simulink model "tir_model"  (Simulink 7.6)
settings: Solver=ode45  StartTime=0.0  StopTime=100  RelTol=1e-3
values from neighbouring files (symbols this model uses):
  ct10 = 27627    [semi_trailer.m]
  ct11 = 0    [semi_trailer.m]
  ct12 = 27627    [semi_trailer.m]
  ct13 = 0    [semi_trailer.m]
  ct14 = 27627    [semi_trailer.m]
  ct15 = 0    [semi_trailer.m]
  ct16 = 27627    [semi_trailer.m]
  ct17 = 0    [semi_trailer.m]
  ct18 = 10000    [semi_trailer.m]
  ct19 = 0    [semi_trailer.m]
  ct2 = 44506    [semi_trailer.m]
  ct20 = 10000    [semi_trailer.m]
  ct21 = 0    [semi_trailer.m]
  ct4 = 44506    [semi_trailer.m]
  ct6 = 44506    [semi_trailer.m]
  ct8 = 44506    [semi_trailer.m]
  dyt = 0.007    [semi_trailer.m]
  kt10 = 967430    [semi_trailer.m]
  kt11 = 2000000    [semi_trailer.m]
  kt12 = 967430    [semi_trailer.m]
  kt13 = 2000000    [semi_trailer.m]
  kt14 = 967430    [semi_trailer.m]
  kt15 = 2000000    [semi_trailer.m]
  kt16 = 967430    [semi_trailer.m]
  kt17 = 2000000    [semi_trailer.m]
  kt18 = 300000    [semi_trailer.m]
  kt19 = 847000    [semi_trailer.m]
  kt2 = 155800    [semi_trailer.m]
  kt20 = 300000    [semi_trailer.m]
  kt21 = 847000    [semi_trailer.m]
  kt3 = 2000000    [semi_trailer.m]
  kt4 = 155800    [semi_trailer.m]
  kt5 = 2000000    [semi_trailer.m]
  kt6 = 155800    [semi_trailer.m]
  kt7 = 2000000    [semi_trailer.m]
  kt8 = 155800    [semi_trailer.m]
  kt9 = 2000000    [semi_trailer.m]
  Lt11 = 4.8    [semi_trailer.m]
  Lt12 = 1.2    [semi_trailer.m]
  Lt13 = 3.6    [semi_trailer.m]
  Lt14 = 1.2    [semi_trailer.m]
  Lt15 = 1.2    [semi_trailer.m]
  Lt16 = 4.134    [semi_trailer.m]
  Lt21 = 4    [semi_trailer.m]
  Lt22 = 0.685    [semi_trailer.m]
  Lt23 = 0.7    [semi_trailer.m]
  Lt24 = 1.2    [semi_trailer.m]
  Lt25 = 1.2    [semi_trailer.m]
  Lt26 = 6.973    [semi_trailer.m]
  mt10 = 520    [semi_trailer.m]
  mt11 = 270    [semi_trailer.m]
  mt12 = 270    [semi_trailer.m]
  mt3 = 270    [semi_trailer.m]
  mt4 = 270    [semi_trailer.m]
  mt5 = 270    [semi_trailer.m]
  mt6 = 270    [semi_trailer.m]
  mt7 = 520    [semi_trailer.m]
  mt8 = 520    [semi_trailer.m]
  mt9 = 520    [semi_trailer.m]
  Vt = 20    [semi_trailer.m]
  wt = 20/dyt    (= 2857.14285714)    [semi_trailer.m]
settings Model: Creator=user  LastModifiedBy=user

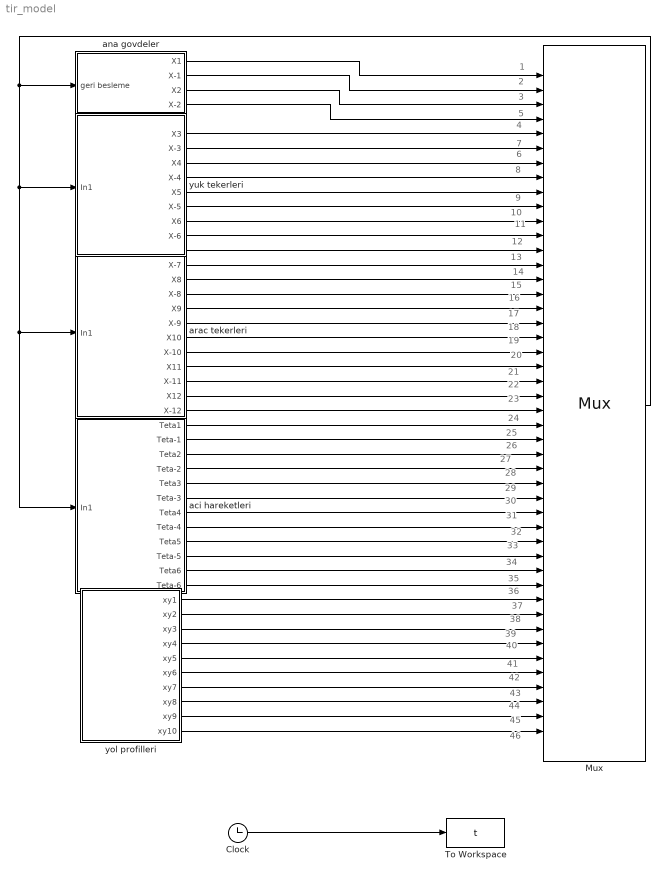
== system tir_model ==
  note: 1
  note: 2
  note: 3
  note: 4
  note: 5
  note: 6
  note: 7
  note: 8
  note: 9
  note: 10
  note: 11
  note: 12
  note: 13
  note: 14
  note: 15
  note: 16
  note: 17
  note: 18
  note: 19
  note: 20
  note: 21
  note: 22
  note: 23
  note: 24
  note: 25
  note: 26
  note: 27
  note: 28
  note: 29
  note: 30
  note: 31
  note: 32
  note: 33
  note: 34
  note: 35
  note: 36
  note: 37
  note: 38
  note: 39
  note: 40
  note: 41
  note: 42
  note: 43
  note: 44
  note: 45
  note: 46
  Clock : Clock
      settings: Decimation=10
  Mux : Mux  Inputs=46
  To Workspace : ToWorkspace  VariableName=t  SampleTime=-1  SaveFormat=Array
  aci hareketleri : Subsystem
  ana govdeler : Subsystem
  arac tekerleri : Subsystem
  yol profilleri : Subsystem
  "yuk tekerleri " : Subsystem
  wires:
  Clock/1 -> To Workspace/1
  "yuk tekerleri "/1(X3) -> Mux/5
  "yuk tekerleri "/2(X-3) -> Mux/6
  "yuk tekerleri "/3(X4) -> Mux/7
  "yuk tekerleri "/4(X-4) -> Mux/8
  "yuk tekerleri "/5(X5) -> Mux/9
  "yuk tekerleri "/6(X-5) -> Mux/10
  "yuk tekerleri "/7(X6) -> Mux/11
  "yuk tekerleri "/8(X-6) -> Mux/12
  arac tekerleri/1(X7) -> Mux/13
  arac tekerleri/2(X-7) -> Mux/14
  arac tekerleri/3(X8) -> Mux/15
  arac tekerleri/4(X-8) -> Mux/16
  arac tekerleri/5(X9) -> Mux/17
  arac tekerleri/6(X-9) -> Mux/18
  arac tekerleri/7(X10) -> Mux/19
  arac tekerleri/8(X-10) -> Mux/20
  arac tekerleri/9(X11) -> Mux/21
  arac tekerleri/10(X-11) -> Mux/22
  arac tekerleri/11(X12) -> Mux/23
  arac tekerleri/12(X-12) -> Mux/24
  aci hareketleri/1(Teta1) -> Mux/25
  aci hareketleri/2(Teta-1) -> Mux/26
  aci hareketleri/3(Teta2) -> Mux/27
  aci hareketleri/4(Teta-2) -> Mux/28
  aci hareketleri/5(Teta3) -> Mux/29
  aci hareketleri/6(Teta-3) -> Mux/30
  aci hareketleri/7(Teta4) -> Mux/31
  aci hareketleri/8(Teta-4) -> Mux/32
  aci hareketleri/9(Teta5) -> Mux/33
  aci hareketleri/10(Teta-5) -> Mux/34
  aci hareketleri/11(Teta6) -> Mux/35
  aci hareketleri/12(Teta-6) -> Mux/36
  Mux/1 -> aci hareketleri/1(In1), arac tekerleri/1(In1), "yuk tekerleri "/1(In1), ana govdeler/1(geri besleme)
  ana govdeler/1(X1) -> Mux/1
  ana govdeler/2(X-1) -> Mux/2
  ana govdeler/3(X2) -> Mux/3
  ana govdeler/4(X-2) -> Mux/4
  yol profilleri/1(xy1) -> Mux/37
  yol profilleri/2(xy2) -> Mux/38
  yol profilleri/3(xy3) -> Mux/39
  yol profilleri/4(xy4) -> Mux/40
  yol profilleri/5(xy5) -> Mux/41
  yol profilleri/6(xy6) -> Mux/42
  yol profilleri/7(xy7) -> Mux/43
  yol profilleri/8(xy8) -> Mux/44
  yol profilleri/9(xy9) -> Mux/45
  yol profilleri/10(xy10) -> Mux/46

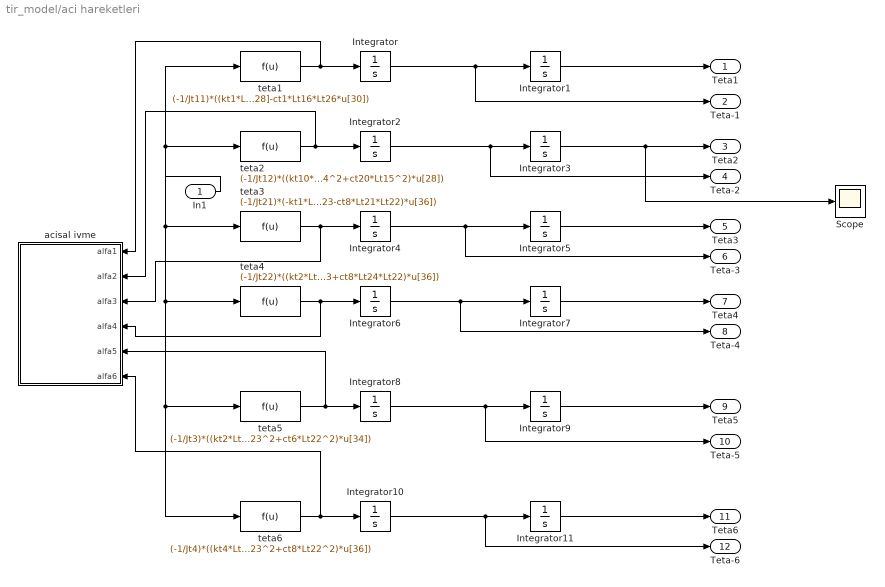
== system tir_model/aci hareketleri ==
  In1 : Inport
  Integrator{,1..11} (12 alike) : Integrator
  Scope : Scope
      settings: SaveName=ScopeData2
  acisal ivme : Subsystem
  teta1 : Fcn  Expr=(-1/Jt11)*((kt1*Lt16+kt10*Lt11+kt12*Lt11+kt14*Lt13+kt16*Lt13-kt18*Lt12-kt20*Lt12)*u[1]+kt1*Lt16*u[3]-kt10*Lt11*u[13]-kt12*Lt11*u[15]-kt14*Lt13*u[17]-kt16*Lt13*u[19]+kt18*Lt12*u[21]+kt20*Lt12*u[23]+(kt1*Lt16^2+kt10*Lt11^2+kt12*Lt11^2+kt14*Lt13^2+kt16*Lt13^2+kt18*Lt12^2+kt20*Lt12^2)*u[25]+(kt10*Lt11*Lt14-kt12*Lt11*Lt15+kt14*Lt13*Lt14-kt16*Lt13*Lt15-kt18*Lt12*Lt14+kt20*Lt12*Lt15)*u[27]-kt1*Lt16*Lt26*u[29]+(ct1*Lt16+ct10*Lt11+ct12*Lt11+ct14*Lt13+ct16*Lt13-ct18*Lt12-ct20*Lt12)*u[2]+ct1*Lt16*u[4]-ct10*Lt11*u[14]-ct12*Lt11*u[16]-ct14*Lt13*u[18]-ct16*Lt13*u[20]+ct18*Lt12*u[22]+ct20*Lt12*u[24]+(ct1*Lt16^2+ct10*Lt11^2+ct12*Lt11^2+ct14*Lt13^2+ct16*Lt13^2+ct18*Lt12^2+ct20*Lt12^2)*u[26]+(ct10*Lt11*Lt14-ct12*Lt11*Lt15+ct14*Lt13*Lt14-ct16*Lt13*Lt15-ct18*Lt12*Lt14+ct20*Lt12*Lt15)*u[28]-ct1*Lt16*Lt26*u[30])
  teta2 : Fcn  Expr=(-1/Jt12)*((kt10*Lt14-kt12*Lt15+kt14*Lt14-kt16*Lt15+kt18*Lt14-kt20*Lt15)*u[1]-kt10*Lt14*u[13]+kt12*Lt15*u[15]-kt14*Lt14*u[17]+kt16*Lt15*u[19]-kt18*Lt14*u[21]+kt20*Lt15*u[23]+(kt10*Lt11*Lt14-kt12*Lt11*Lt15+kt14*Lt13*Lt14-kt16*Lt13*Lt15-kt18*Lt12*Lt14+kt20*Lt12*Lt15)*u[25]+(kt10*Lt14^2+kt12*Lt15^2+kt14*Lt14^2+kt16*Lt15^2+kt18*Lt14^2+kt20*Lt15^2)*u[27]+(ct10*Lt14-ct12*Lt15+ct14*Lt14-ct16*Lt15+ct18*Lt14-ct20*Lt15)*u[2]-ct10*Lt14*u[14]+ct12*Lt15*u[16]-ct14*Lt14*u[18]+ct16*Lt15*u[20]-ct18*Lt14*u[22]+ct20*Lt15*u[24]+(ct10*Lt11*Lt14-ct12*Lt11*Lt15+ct14*Lt13*Lt14-ct16*Lt13*Lt15-ct18*Lt12*Lt14+ct20*Lt12*Lt15)*u[26]+(ct10*Lt14^2+ct12*Lt15^2+ct14*Lt14^2+ct16*Lt15^2+ct18*Lt14^2+ct20*Lt15^2)*u[28])
  teta3 : Fcn  Expr=(-1/Jt21)*(-kt1*Lt26*u[1]+(-kt1*Lt26+kt2*Lt21+kt4*Lt21+kt6*Lt21+kt8*Lt21)*u[3]-kt2*Lt21*u[5]-kt4*Lt21*u[7]-kt6*Lt21*u[9]-kt8*Lt21*u[11]-kt1*Lt16*Lt26*u[25]+(kt1*Lt26^2+kt2*Lt21^2+kt4*Lt21^2+kt6*Lt21^2+kt8*Lt21^2)*u[29]+(kt2*Lt21*Lt24-kt4*Lt21*Lt25+kt6*Lt21*Lt24-kt8*Lt21*Lt25)*u[31]+(kt2*Lt21*Lt23-kt6*Lt21*Lt22)*u[33]+(kt4*Lt21*Lt23-kt8*Lt21*Lt22)*u[35]-ct1*Lt26*u[2]+(-ct1*Lt26+ct2*Lt21+ct4*Lt21+ct6*Lt21+ct8*Lt21)*u[4]-ct2*Lt21*u[6]-ct4*Lt21*u[8]-ct6*Lt21*u[10]-ct8*Lt21*u[12]-ct1*Lt16*Lt26*u[26]+(ct1*Lt26^2+ct2*Lt21^2+ct4*Lt21^2+ct6*Lt21^2+ct8*Lt21^2)*u[30]+(ct2*Lt21*Lt24-ct4*Lt21*Lt25+ct6*Lt21*Lt24-ct8*Lt21*Lt25)*u[32]+(ct2*Lt21*Lt23-ct6*Lt21*Lt22)*u[34]+(ct4*Lt21*Lt23-ct8*Lt21*Lt22)*u[36])
  teta4 : Fcn  Expr=(-1/Jt22)*((kt2*Lt24-kt4*Lt25+kt6*Lt24-kt8*Lt25)*u[3]-kt2*Lt24*u[5]+kt4*Lt25*u[7]-kt6*Lt24*u[9]+kt8*Lt25*u[11] +(kt2*Lt21*Lt24-kt4*Lt21*Lt25+kt6*Lt21*Lt24-kt8*Lt21*Lt25)*u[29]+(kt2*Lt24^2+kt4*Lt25^2+kt6*Lt24^2+kt8*Lt25^2)*u[31]+(kt2*Lt24*Lt23-kt6*Lt24*Lt22)*u[33]+(-kt4*Lt25*Lt23+kt8*Lt24*Lt22)*u[35]+(ct2*Lt24-ct4*Lt25+ct6*Lt24-ct8*Lt25)*u[4]-ct2*Lt24*u[6]+ct4*Lt25*u[8]-ct6*Lt24*u[10]+ct8*Lt25*u[12]+(ct2*Lt21*Lt24-ct4*Lt21*Lt25+ct6*Lt21*Lt24-ct8*Lt21*Lt25)*u[30]+(ct2*Lt24^2+ct4*Lt25^2+ct6*Lt24^2+ct8*Lt25^2)*u[32]+(ct2*Lt24*Lt23-ct6*Lt24*Lt22)*u[34]+(-ct4*Lt25*Lt23+ct8*Lt24*Lt22)*u[36])
  teta5 : Fcn  Expr=(-1/Jt3)*((kt2*Lt23-kt6*Lt22)*u[3]-kt2*Lt23*u[5]+kt6*Lt22*u[9]+(kt2*Lt23*Lt21-kt6*Lt22*Lt21)*u[29]+(kt2*Lt23*Lt24-kt6*Lt22*Lt24)*u[31]+(kt2*Lt23^2+kt6*Lt22^2)*u[33]+(ct2*Lt23-ct6*Lt22)*u[4]-ct2*Lt23*u[6]+ct6*Lt22*u[10]+(ct2*Lt23*Lt21-ct6*Lt22*Lt21)*u[30]+(ct2*Lt23*Lt24-ct6*Lt22*Lt24)*u[32]+(ct2*Lt23^2+ct6*Lt22^2)*u[34])
  teta6 : Fcn  Expr=(-1/Jt4)*((kt4*Lt23-kt8*Lt22)*u[3]-kt4*Lt23*u[7]+kt8*Lt22*u[11]+(kt4*Lt23*Lt21-kt8*Lt22*Lt21)*u[29]+(-kt4*Lt23*Lt25+kt8*Lt22*Lt25)*u[31]+(kt4*Lt23^2+kt8*Lt22^2)*u[35]+(ct4*Lt23-ct8*Lt22)*u[4]-ct4*Lt23*u[8]+ct8*Lt22*u[12]+(ct4*Lt23*Lt21-ct8*Lt22*Lt21)*u[30]+(-ct4*Lt23*Lt25+ct8*Lt22*Lt25)*u[32]+(ct4*Lt23^2+ct8*Lt22^2)*u[36])
  Teta1 : Outport
  Teta-1 : Outport  Port=2
  Teta2 : Outport  Port=3
  Teta-2 : Outport  Port=4
  Teta3 : Outport  Port=5
  Teta-3 : Outport  Port=6
  Teta4 : Outport  Port=7
  Teta-4 : Outport  Port=8
  Teta5 : Outport  Port=9
  Teta-5 : Outport  Port=10
  Teta6 : Outport  Port=11
  Teta-6 : Outport  Port=12
  wires:
  Integrator10/1 -> Integrator11/1, Teta-6/1
  teta6/1 -> Integrator10/1, acisal ivme/6(alfa6)
  Integrator8/1 -> Integrator9/1, Teta-5/1
  teta5/1 -> Integrator8/1, acisal ivme/5(alfa5)
  In1/1 -> teta1/1, teta2/1, teta6/1, teta5/1, teta4/1, teta3/1
  Integrator2/1 -> Integrator3/1, Teta-2/1
  teta2/1 -> Integrator2/1, acisal ivme/2(alfa2)
  Integrator/1 -> Integrator1/1, Teta-1/1
  teta1/1 -> Integrator/1, acisal ivme/1(alfa1)
  Integrator6/1 -> Integrator7/1, Teta-4/1
  teta4/1 -> Integrator6/1, acisal ivme/4(alfa4)
  Integrator4/1 -> Integrator5/1, Teta-3/1
  teta3/1 -> Integrator4/1, acisal ivme/3(alfa3)
  Integrator1/1 -> Teta1/1
  Integrator3/1 -> Teta2/1, Scope/1
  Integrator5/1 -> Teta3/1
  Integrator7/1 -> Teta4/1
  Integrator9/1 -> Teta5/1
  Integrator11/1 -> Teta6/1

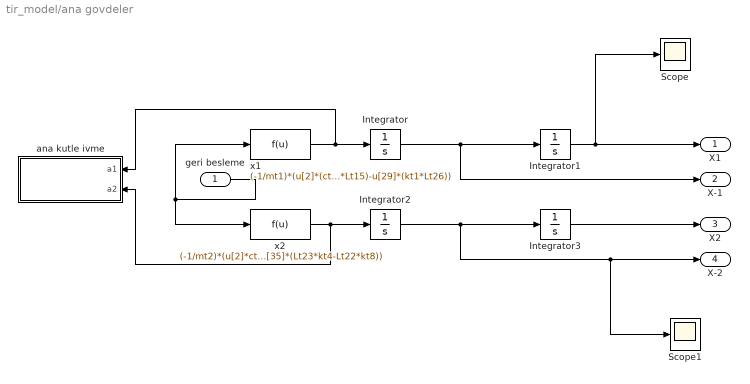
== system tir_model/ana govdeler ==
  geri besleme : Inport
  Integrator{,1..3} (4 alike) : Integrator
  Scope : Scope
  Scope1 : Scope
  ana kutle ivme : Subsystem
  x1 : Fcn  Expr=(-1/mt1)*(u[2]*(ct1+ct10+ct12+ct14+ct16+ct18+ct20)+u[4]*ct1-u[14]*ct10-u[16]*ct12-u[18]*ct14-u[20]*ct16-u[22]*ct18-u[24]*ct20+u[26]*(ct1*Lt16+ct10*Lt11+ct12*Lt11+ct14*Lt13+ct16*Lt13-ct18*Lt12-ct20*Lt12)+ u[28]*(ct10*Lt14-ct12*Lt15+ct14*Lt14-ct16*Lt15+ct18*Lt14-ct20*Lt15)-u[30]*(ct1*Lt26)+ u[1]*(kt1+kt10+kt12+kt14+kt16+kt18+kt20)+u[3]*kt1-u[13]*kt10-u[15]*kt12-u[17]*kt14-u[19]*kt16-u[21]*kt18-u[23]*kt20+u[25]*(kt1*Lt16+kt10*Lt11+kt12*Lt11+kt14*Lt13+kt16*Lt13-kt18*Lt12-kt20*Lt12)+ u[27]*(kt10*Lt14-kt12*Lt15+kt14*Lt14-kt16*Lt15+kt18*Lt14-kt20*Lt15)-u[29]*(kt1*Lt26))
  x2 : Fcn  Expr=(-1/mt2)*(u[2]*ct1+u[4]*(ct1+ct2+ct4+ct6+ct8)-u[6]*ct2-u[8]*ct4-u[10]*ct6-u[12]*ct8 +u[26]*(ct1*Lt16)+ u[30]*(-ct1*Lt26+(ct2+ct4+ct6+ct8)*Lt21)+ u[32]*(Lt24*ct2-Lt25*ct4+Lt24*ct6-Lt25*ct8)+u[34]*(Lt23*ct2-Lt22*ct6)+u[36]*(Lt23*ct4-Lt22*ct8) + u[1]*kt1+u[3]*(kt1+kt2+kt4+kt6+kt8)-u[5]*kt2-u[7]*kt4-u[9]*kt6-u[11]*kt8 +u[25]*(kt1*Lt16)+ u[29]*(-kt1*Lt26+(kt2+kt4+kt6+kt8)*Lt21)+ u[31]*(Lt24*kt2-Lt25*kt4+Lt24*kt6-Lt25*kt8)+u[33]*(Lt23*kt2-Lt22*kt6)+u[35]*(Lt23*kt4-Lt22*kt8))
  X1 : Outport
  X-1 : Outport  Port=2
  X2 : Outport  Port=3
  X-2 : Outport  Port=4
  wires:
  x1/1 -> Integrator/1, ana kutle ivme/1(a1)
  Integrator/1 -> Integrator1/1, X-1/1
  x2/1 -> Integrator2/1, ana kutle ivme/2(a2)
  Integrator2/1 -> Integrator3/1, X-2/1, Scope1/1
  geri besleme/1 -> x1/1, x2/1
  Integrator1/1 -> X1/1, Scope/1
  Integrator3/1 -> X2/1

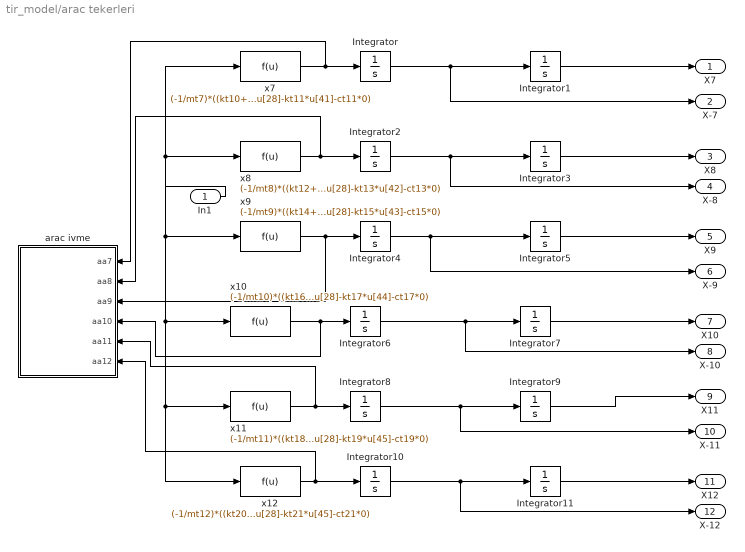
== system tir_model/arac tekerleri ==
  In1 : Inport
  Integrator{,1..11} (12 alike) : Integrator
  arac ivme : Subsystem
  x10 : Fcn  Expr=(-1/mt10)*((kt16+kt17)*u[19]+(ct16+ct17)*u[20]-kt16*u[1]-Lt13*kt16*u[25]+Lt15*kt16*u[27]-ct16*u[2]-Lt13*ct16*u[26]+Lt15*ct16*u[28]-kt17*u[44]-ct17*0)
  x11 : Fcn  Expr=(-1/mt11)*((kt18+kt19)*u[21]+(ct18+ct19)*u[22]-kt18*u[1]+Lt12*kt18*u[25]-Lt14*kt18*u[27]-ct18*u[2]+Lt12*ct18*u[26]-Lt14*ct18*u[28]-kt19*u[45]-ct19*0)
  x12 : Fcn  Expr=(-1/mt12)*((kt20+kt21)*u[23]+(ct20+ct21)*u[24]-kt20*u[1]+Lt12*kt20*u[25]+Lt15*kt20*u[27]-ct20*u[2]+Lt12*ct20*u[26]+Lt15*ct20*u[28]-kt21*u[45]-ct21*0)
  x7 : Fcn  Expr=(-1/mt7)*((kt10+kt11)*u[13]+(ct10+ct11)*u[14]-kt10*u[1]-Lt11*kt10*u[25]-Lt14*kt10*u[27]-ct10*u[2]-Lt11*ct10*u[26]-Lt14*ct10*u[28]-kt11*u[41]-ct11*0)
  x8 : Fcn  Expr=(-1/mt8)*((kt12+kt13)*u[15]+(ct12+ct13)*u[16]-kt12*u[1]-Lt11*kt12*u[25]+Lt15*kt12*u[27]-ct12*u[2]-Lt11*ct12*u[26]+Lt15*ct12*u[28]-kt13*u[42]-ct13*0)
  x9 : Fcn  Expr=(-1/mt9)*((kt14+kt15)*u[17]+(ct14+ct15)*u[18]-kt14*u[1]-Lt13*kt14*u[25]-Lt14*kt14*u[27]-ct14*u[2]-Lt13*ct14*u[26]-Lt14*ct14*u[28]-kt15*u[43]-ct15*0)
  X7 : Outport
  X-7 : Outport  Port=2
  X8 : Outport  Port=3
  X-8 : Outport  Port=4
  X9 : Outport  Port=5
  X-9 : Outport  Port=6
  X10 : Outport  Port=7
  X-10 : Outport  Port=8
  X11 : Outport  Port=9
  X-11 : Outport  Port=10
  X12 : Outport  Port=11
  X-12 : Outport  Port=12
  wires:
  x9/1 -> Integrator4/1, arac ivme/3(aa9)
  Integrator4/1 -> Integrator5/1, X-9/1
  x10/1 -> Integrator6/1, arac ivme/4(aa10)
  Integrator6/1 -> Integrator7/1, X-10/1
  x7/1 -> Integrator/1, arac ivme/1(aa7)
  Integrator/1 -> Integrator1/1, X-7/1
  x8/1 -> Integrator2/1, arac ivme/2(aa8)
  Integrator2/1 -> Integrator3/1, X-8/1
  In1/1 -> x9/1, x10/1, x11/1, x12/1, x8/1, x7/1
  x11/1 -> Integrator8/1, arac ivme/5(aa11)
  Integrator8/1 -> Integrator9/1, X-11/1
  x12/1 -> Integrator10/1, arac ivme/6(aa12)
  Integrator10/1 -> Integrator11/1, X-12/1
  Integrator1/1 -> X7/1
  Integrator3/1 -> X8/1
  Integrator5/1 -> X9/1
  Integrator7/1 -> X10/1
  Integrator9/1 -> X11/1
  Integrator11/1 -> X12/1

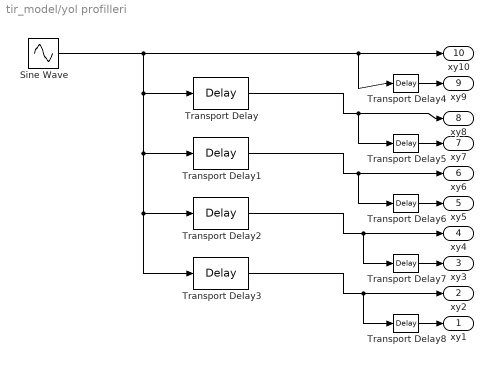
== system tir_model/yol profilleri ==
  Sine Wave : Sin  Amplitude=dyt  Frequency=wt  SampleTime=0
  Transport Delay : TransportDelay  DelayTime=(Lt12+Lt13)/Vt
  Transport Delay1 : TransportDelay  DelayTime=(Lt12+Lt11)/Vt
  Transport Delay2 : TransportDelay  DelayTime=(Lt12+Lt16+Lt26+Lt21-Lt22)/Vt
  Transport Delay3 : TransportDelay  DelayTime=(Lt12+Lt16+Lt26+Lt21+Lt23)/Vt
  Transport Delay{4..8} (5 alike) : TransportDelay  DelayTime=0.001
  xy1 : Outport
  xy2 : Outport  Port=2
  xy3 : Outport  Port=3
  xy4 : Outport  Port=4
  xy5 : Outport  Port=5
  xy6 : Outport  Port=6
  xy7 : Outport  Port=7
  xy8 : Outport  Port=8
  xy9 : Outport  Port=9
  xy10 : Outport  Port=10
  wires:
  Sine Wave/1 -> Transport Delay2/1, Transport Delay3/1, Transport Delay1/1, Transport Delay/1, xy10/1, Transport Delay4/1
  Transport Delay/1 -> xy8/1, Transport Delay5/1
  Transport Delay1/1 -> xy6/1, Transport Delay6/1
  Transport Delay2/1 -> xy4/1, Transport Delay7/1
  Transport Delay3/1 -> xy2/1, Transport Delay8/1
  Transport Delay4/1 -> xy9/1
  Transport Delay5/1 -> xy7/1
  Transport Delay6/1 -> xy5/1
  Transport Delay7/1 -> xy3/1
  Transport Delay8/1 -> xy1/1

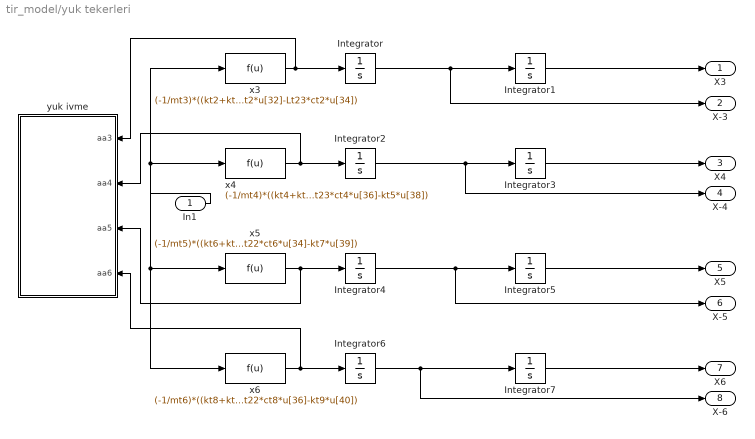
== system tir_model/yuk tekerleri  ==
  In1 : Inport
  Integrator{,1..7} (8 alike) : Integrator
  x3 : Fcn  Expr=(-1/mt3)*((kt2+kt3)*u[5]+(ct2)*u[6]-kt2*u[3]-Lt21*kt2*u[29]-Lt24*kt2*u[31]-Lt23*kt2*u[33]-ct2*u[4]-Lt21*ct2*u[30]-Lt24*ct2*u[32]-Lt23*ct2*u[34])
  x4 : Fcn  Expr=(-1/mt4)*((kt4+kt5)*u[7]+(ct4)*u[8]-kt4*u[3]-Lt21*kt4*u[29]+Lt25*kt4*u[31]-Lt23*kt4*u[35]-ct4*u[4]-Lt21*ct4*u[30]+Lt25*ct4*u[32]-Lt23*ct4*u[36]-kt5*u[38])
  x5 : Fcn  Expr=(-1/mt5)*((kt6+kt7)*u[9]+(ct6)*u[10]-kt6*u[3]-Lt21*kt6*u[29]-Lt24*kt6*u[31]+Lt22*kt6*u[33]-ct6*u[4]-Lt21*ct6*u[30]-Lt24*ct6*u[32]+Lt22*ct6*u[34]-kt7*u[39])
  x6 : Fcn  Expr=(-1/mt6)*((kt8+kt9)*u[11]+(ct8)*u[12]-kt8*u[3]-Lt21*kt8*u[29]+Lt25*kt8*u[31]+Lt22*kt8*u[35]-ct8*u[4]-Lt21*ct8*u[30]+Lt25*ct8*u[32]+Lt22*ct8*u[36]-kt9*u[40])
  yuk ivme : Subsystem
  X3 : Outport
  X-3 : Outport  Port=2
  X4 : Outport  Port=3
  X-4 : Outport  Port=4
  X5 : Outport  Port=5
  X-5 : Outport  Port=6
  X6 : Outport  Port=7
  X-6 : Outport  Port=8
  wires:
  In1/1 -> x3/1, x4/1, x5/1, x6/1
  Integrator2/1 -> Integrator3/1, X-4/1
  x4/1 -> Integrator2/1, yuk ivme/2(aa4)
  Integrator/1 -> Integrator1/1, X-3/1
  x3/1 -> Integrator/1, yuk ivme/1(aa3)
  Integrator6/1 -> Integrator7/1, X-6/1
  x6/1 -> Integrator6/1, yuk ivme/4(aa6)
  Integrator4/1 -> Integrator5/1, X-5/1
  x5/1 -> Integrator4/1, yuk ivme/3(aa5)
  Integrator1/1 -> X3/1
  Integrator3/1 -> X4/1
  Integrator5/1 -> X5/1
  Integrator7/1 -> X6/1

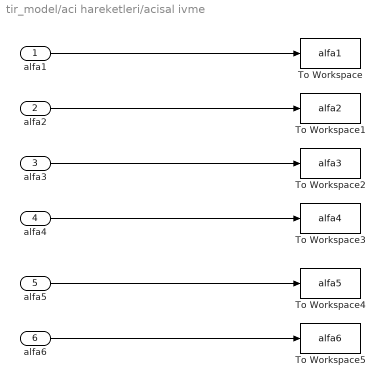
== system tir_model/aci hareketleri/acisal ivme ==
  alfa1 : Inport
  alfa2 : Inport  Port=2
  alfa3 : Inport  Port=3
  alfa4 : Inport  Port=4
  alfa5 : Inport  Port=5
  alfa6 : Inport  Port=6
  To Workspace : ToWorkspace  VariableName=alfa1  SampleTime=-1  SaveFormat=Array
  To Workspace1 : ToWorkspace  VariableName=alfa2  SampleTime=-1  SaveFormat=Array
  To Workspace2 : ToWorkspace  VariableName=alfa3  SampleTime=-1  SaveFormat=Array
  To Workspace3 : ToWorkspace  VariableName=alfa4  SampleTime=-1  SaveFormat=Array
  To Workspace4 : ToWorkspace  VariableName=alfa5  SampleTime=-1  SaveFormat=Array
  To Workspace5 : ToWorkspace  VariableName=alfa6  SampleTime=-1  SaveFormat=Array
  wires:
  alfa1/1 -> To Workspace/1
  alfa2/1 -> To Workspace1/1
  alfa3/1 -> To Workspace2/1
  alfa4/1 -> To Workspace3/1
  alfa5/1 -> To Workspace4/1
  alfa6/1 -> To Workspace5/1

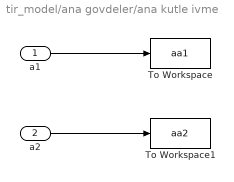
== system tir_model/ana govdeler/ana kutle ivme ==
  a1 : Inport
  a2 : Inport  Port=2
  To Workspace : ToWorkspace  VariableName=aa1  SampleTime=-1  SaveFormat=Array
  To Workspace1 : ToWorkspace  VariableName=aa2  SampleTime=-1  SaveFormat=Array
  wires:
  a1/1 -> To Workspace/1
  a2/1 -> To Workspace1/1

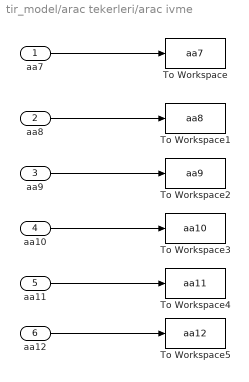
== system tir_model/arac tekerleri/arac ivme ==
  aa7 : Inport
  aa8 : Inport  Port=2
  aa9 : Inport  Port=3
  aa10 : Inport  Port=4
  aa11 : Inport  Port=5
  aa12 : Inport  Port=6
  To Workspace : ToWorkspace  VariableName=aa7  SampleTime=-1  SaveFormat=Array
  To Workspace1 : ToWorkspace  VariableName=aa8  SampleTime=-1  SaveFormat=Array
  To Workspace2 : ToWorkspace  VariableName=aa9  SampleTime=-1  SaveFormat=Array
  To Workspace3 : ToWorkspace  VariableName=aa10  SampleTime=-1  SaveFormat=Array
  To Workspace4 : ToWorkspace  VariableName=aa11  SampleTime=-1  SaveFormat=Array
  To Workspace5 : ToWorkspace  VariableName=aa12  SampleTime=-1  SaveFormat=Array
  wires:
  aa7/1 -> To Workspace/1
  aa8/1 -> To Workspace1/1
  aa9/1 -> To Workspace2/1
  aa10/1 -> To Workspace3/1
  aa11/1 -> To Workspace4/1
  aa12/1 -> To Workspace5/1

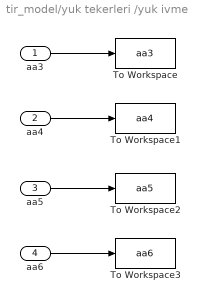
== system tir_model/yuk tekerleri /yuk ivme ==
  aa3 : Inport
  aa4 : Inport  Port=2
  aa5 : Inport  Port=3
  aa6 : Inport  Port=4
  To Workspace : ToWorkspace  VariableName=aa3  SampleTime=-1  SaveFormat=Array
  To Workspace1 : ToWorkspace  VariableName=aa4  SampleTime=-1  SaveFormat=Array
  To Workspace2 : ToWorkspace  VariableName=aa5  SampleTime=-1  SaveFormat=Array
  To Workspace3 : ToWorkspace  VariableName=aa6  SampleTime=-1  SaveFormat=Array
  wires:
  aa3/1 -> To Workspace/1
  aa4/1 -> To Workspace1/1
  aa5/1 -> To Workspace2/1
  aa6/1 -> To Workspace3/1
